simulink model "hdl_model_1"  (R2015b)
settings: Solver=VariableStepAuto  StartTime=0.0  StopTime=400  RelTol=1e-3
model workspace (MAT data in the model file):
  BUCKET_NUMBER = Simulink.Parameter
  BUCKET_NUMBER.Value = 2708
  BUCKET_NUMBER.DataType = 'uint16'
  BUCKET_NUMBER.Units = 'auto'
  BUNCH_NUM = Simulink.Parameter
  BUNCH_NUM.Value = 50
  BUNCH_NUM.DataType = 'uint16'
  BUNCH_NUM.Units = 'auto'
  BUNCH_SPACE = Simulink.Parameter
  BUNCH_SPACE.Value = 4
  BUNCH_SPACE.DataType = 'uint16'
  BUNCH_SPACE.Units = 'auto'
  SYS_DEL = Simulink.Parameter
  SYS_DEL.Value = 9
  SYS_DEL.DataType = 'uint8'
  SYS_DEL.Units = 'auto'
libraries: simulink x6, hdlsllib x2
settings Model: Creator=koprek_w  LastModifiedBy=koprek_w

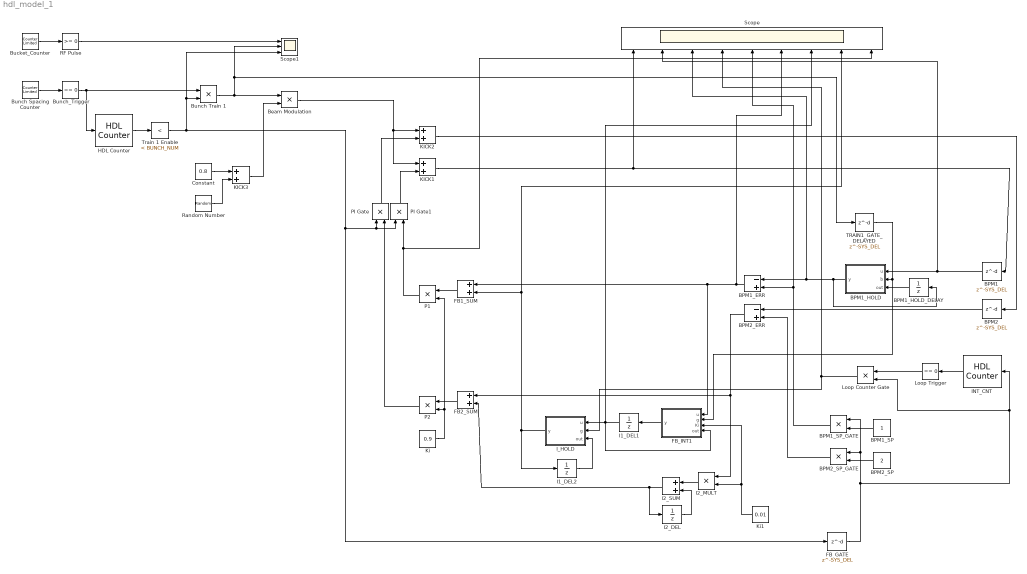
== system hdl_model_1 ==
  BPM1 : Delay  DelayLength=SYS_DEL
  BPM1_ERR : Sum  Inputs=-+
  BPM1_HOLD : MATLAB Function  TreatAsAtomicUnit=on
  BPM1_HOLD_DELAY : UnitDelay  SampleTime=-1
  BPM1_SP : Constant  SampleTime=-1
  BPM1_SP_GATE : Product
  BPM2 : Delay  DelayLength=SYS_DEL
  BPM2_ERR : Sum  Inputs=-+
  BPM2_SP : Constant  Value=2
  BPM2_SP_GATE : Product
  Beam Modulation : Product
  Bucket_Counter : simulink/Sources/Counter Limited  uplimit=BUCKET_NUMBER-1  tsamp=1
  Bunch Spacing Counter : simulink/Sources/Counter Limited  uplimit=BUNCH_SPACE-1  tsamp=1
  Bunch Train 1 : Product
  Bunch_Trigger : simulink/Logic and Bit Operations/Compare To Constant  relop===  const=0  OutDataTypeStr=boolean
  Constant : Constant  Value=0.8  SampleTime=-1
  FB1_SUM : Sum
  FB2_SUM : Sum
  FB_GATE : Delay  DelayLength=SYS_DEL
  FB_INT1 : MATLAB Function  TreatAsAtomicUnit=on
  HDL Counter : hdlsllib/HDL Operations/HDL Counter  CountType=Free running  CountInit=0  CountStep=1  CountMax=25  CountFromType=Initial value  CountFrom=0  CountResetPort=off  CountLoadPort=off  CountEnbPort=on  CountDirPort=off  CountDataType=Unsigned  CountWordLen=16  CountFracLen=0  CountSampTime=1
  I1_DEL1 : UnitDelay  SampleTime=-1
  I1_DEL2 : UnitDelay  SampleTime=-1
  I2_DEL : UnitDelay  SampleTime=-1
  I2_MULT : Product
  I2_SUM : Sum
  INT_CNT : hdlsllib/HDL Operations/HDL Counter  CountType=Count limited  CountInit=0  CountStep=1  CountMax=11  CountFromType=Initial value  CountFrom=0  CountResetPort=off  CountLoadPort=off  CountEnbPort=on  CountDirPort=off  CountDataType=Unsigned  CountWordLen=16  CountFracLen=0  CountSampTime=1
  I_HOLD : MATLAB Function  TreatAsAtomicUnit=on
  KICK1 : Sum
  KICK2 : Sum
  KICK3 : Sum
  Ki : Constant  Value=0.9
  Ki1 : Constant  Value=0.01
  Loop Counter Gate : Product
  Loop Trigger : simulink/Logic and Bit Operations/Compare To Constant  relop===  const=0  OutDataTypeStr=boolean
  P1 : Product
  P2 : Product
  PI Gate : Product
  PI Gate1 : Product
  RF Pulse : simulink/Logic and Bit Operations/Compare To Constant  relop=>=  const=0  OutDataTypeStr=boolean
  Random Number : RandomNumber  Variance=0.001  SampleTime=1
  Scope : Scope  NumInputPorts=9
  Scope1 : Scope  NumInputPorts=3
  TRAIN1_GATE_DELAYED : Delay  DelayLength=SYS_DEL
  Train 1 Enable : simulink/Logic and Bit Operations/Compare To Constant  relop=<  const=BUNCH_NUM  OutDataTypeStr=boolean
  wires:
  KICK1/1 -> BPM1/1, Scope/1
  KICK2/1 -> BPM2/1
  Ki/1 -> P1/2, P2/2
  BPM1/1 -> Scope/2, BPM1_HOLD/1(u)
  BPM2/1 -> BPM2_ERR/1
  BPM1_ERR/1 -> FB_INT1/1(u), FB1_SUM/1, Scope/6
  BPM2_ERR/1 -> I2_MULT/1, FB2_SUM/1
  FB_GATE/1 -> Loop Counter Gate/2, INT_CNT/1, BPM1_SP_GATE/1, BPM2_SP_GATE/1
  BPM1_SP_GATE/1 -> BPM1_ERR/2, Scope/5
  BPM2_SP_GATE/1 -> BPM2_ERR/2
  BPM2_SP/1 -> BPM2_SP_GATE/2
  BPM1_SP/1 -> BPM1_SP_GATE/2
  I2_MULT/1 -> I2_SUM/1
  Ki1/1 -> FB_INT1/3(Ki), I2_MULT/2
  I2_DEL/1 -> I2_SUM/2
  FB1_SUM/1 -> P1/1
  FB2_SUM/1 -> P2/1
  I2_SUM/1 -> FB2_SUM/2, I2_DEL/1
  Bucket_Counter/1 -> RF Pulse/1
  Bunch Spacing Counter/1 -> Bunch_Trigger/1
  Bunch_Trigger/1 -> Bunch Train 1/1, HDL Counter/1
  RF Pulse/1 -> Scope1/1
  HDL Counter/1 -> Train 1 Enable/1
  Train 1 Enable/1 -> FB_GATE/1, PI Gate1/1, PI Gate/1, Scope1/3, Bunch Train 1/2
  Bunch Train 1/1 -> Scope1/2, TRAIN1_GATE_DELAYED/1, Beam Modulation/1
  P2/1 -> PI Gate/2
  PI Gate/1 -> KICK2/2
  P1/1 -> Scope/9, PI Gate1/2
  PI Gate1/1 -> KICK1/2
  Beam Modulation/1 -> KICK1/1, KICK2/1
  I_HOLD/1(y) -> Scope/8, FB1_SUM/2, I1_DEL2/1
  Constant/1 -> KICK3/1
  Random Number/1 -> KICK3/2
  KICK3/1 -> Beam Modulation/2
  BPM1_HOLD/1(y) -> BPM1_ERR/1, Scope/3, BPM1_HOLD_DELAY/1
  TRAIN1_GATE_DELAYED/1 -> BPM1_HOLD/2(b), FB_INT1/2(g)
  BPM1_HOLD_DELAY/1 -> BPM1_HOLD/3(out)
  INT_CNT/1 -> Loop Trigger/1
  Loop Trigger/1 -> Loop Counter Gate/1
  Loop Counter Gate/1 -> I_HOLD/2(g), Scope/4
  I1_DEL1/1 -> FB_INT1/4(out), Scope/7, I_HOLD/1(u)
  I1_DEL2/1 -> I_HOLD/3(out)
  FB_INT1/1(y) -> I1_DEL1/1

== matlab function hdl_model_1/BPM1_HOLD ==
  data: u input; y output; b input; out input
function y = fcn(u, b, out)
%#codegen

if b
  y = u ;
else
  y = out;
end

== matlab function hdl_model_1/I_HOLD ==
  data: u input; y output; g input; out input
function y = fcn(u, g, out)
%#codegen

% BS       Ki        INT-CNT
%  1       1/9       FB_DEL-1
%  2       1/5       FB_DEL
%  3       1/3       FB_DEL-1
%  4       1/3       FB_DEL+2



if g
  y = u ;
else
  y = out;
end

== matlab function hdl_model_1/FB_INT1 ==
  data: u input; y output; g input; Ki input; out input
function y = fcn(u, g, Ki, out)
%#codegen

if g
  y = Ki*u + out ;
else
  y = out;
end
